simulink model "GRU_DataGen"  (R2024b)
settings: Solver=ode4  StartTime=0.0  StopTime=34  FixedStep=0.01  RelTol=1e-3
PreLoadFcn:
  | preloadfcn_v2
model workspace (MAT data in the model file):
  db_rt.A = [1 1 1 1 1 1 1 1 1 1 1 1 ... (55440 elements, 11x15x21x4x4)]
  db_rt.B = [0 0 0 0 0 0 0 0 -1.08359632143e-09 -1.08356536573e-09 -1.08354493529e-09 0 ... (27720 elements, 11x15x21x4x2)]
  db_rt.C = [1 1 1 1 1 1 1 1 1 1 1 1 ... (55440 elements, 11x15x21x4x4)]
  db_rt.D = [0 0 0 0 0 0 0 0 0 0 0 0 ... (27720 elements, 11x15x21x4x2)]
  db_rt.E = [3.5162966917e-06 3.51629595104e-06 2.9967648165e-06 2.99676418585e-06 2.9967635552e-06 2.99676229391e-06 2.99676040198e-06 2.99675567214e-06 4.11715267907e-06 4.11708414824e-06 4.11704028806e-06 3.00600683278e-06 ... (13860 elements, 11x15x21x4)]
  db_rt.grid.V = [0.02; 0.04; 0.06; 0.08; 0.1; 0.14; 0.2; 0.35; 0.6; 1; 1.2]
  db_rt.grid.W = [-1.2; -1.02857142857; -0.857142857143; -0.685714285714; -0.514285714286; -0.342857142857; -0.171428571429; 0; 0.171428571429; 0.342857142857; 0.514285714286; 0.685714285714; 0.857142857143; 1.02857142857; 1.2]
  db_rt.grid.T = [-0.174532925199; -0.157079632679; -0.13962634016; -0.12217304764; -0.10471975512; -0.0872664625997; -0.0698131700798; -0.0523598775598; -0.0349065850399; -0.0174532925199; 0; 0.0174532925199; 0.0349065850399; 0.0523598775598; 0.0698131700798; 0.0872664625997; 0.10471975512; 0.12217304764; 0.13962634016; 0.157079632679; 0.174532925199]
  db_rt.Ts = 0.01
  db_rt.nx = 4
  db_rt.nu = 2
  db_rt.ny = 4
  db_rt.nd = 1
  db_rt.Nv = 11
  db_rt.Nw = 15
  db_rt.Nt = 21
  env_paths.root = 'E:\Matlab\Simulink\S-Function_16'
  env_paths.data = 'E:\Matlab\Simulink\S-Function_16\data'
  env_paths.models = 'E:\Matlab\Simulink\S-Function_16\data\models'
  env_paths.paths = 'E:\Matlab\Simulink\S-Function_16\data\paths'
  env_paths.gru = 'E:\Matlab\Simulink\S-Function_16\data\gru'
  env_paths.results.root = 'E:\Matlab\Simulink\S-Function_16\results'
  env_paths.results.simulink = 'E:\Matlab\Simulink\S-Function_16\results\simulink'
  env_paths.results.closed_loop = 'E:\Matlab\Simulink\S-Function_16\results\closed_loop'
  env_paths.results.paths = 'E:\Matlab\Simulink\S-Function_16\results\paths'
  env_paths.results.gru_logs = 'E:\Matlab\Simulink\S-Function_16\results\gru\sim'
  ff_rt.m = 200
  ff_rt.g = 9.81
  ff_rt.c_r = 0.015
  ff_rt.rho = 1.225
  ff_rt.CdA = 0.5
  params.Ts = 0.01
  params.mass = 200
  params.L = 2
  params.W = 0.8
  params.h_cg = 0.5
  params.Lf = 1
  params.Lr = 1
  params.Iz = 16.67
  params.wheel_radius = 0.15
  params.wheel_mass = 1.2
  params.wheel_inertia = 0.0135
  params.motor_torque_constant = 1.21
  params.motor_inertia = 0.00177
  params.motor_current_limit = 9
  params.gear_ratio = 10
  params.gear_efficiency = 0.9
  params.current_limit = 9
  params.steering_time_constant = 0.08
  params.max_steering_angle = 1.57079632679
  params.max_steering_rate = 0.523598775598
  params.max_acceleration = 1
  params.rolling_resistance = 0.015
  params.friction_coefficient = 0.8
  params.air_density = 1.225
  params.drag_coefficient_area = 0.5
  params.gravity = 9.81
  params.front_cornering_stiffness = 300
  params.rear_cornering_stiffness = 300
  params.enable_noise = 0
  params.current_noise_std = 0.2
  params.wheel_speed_noise_std = 0.5
  params.disturbance_noise_std = 3
  params.random_seed = 42
  params.v_noise_std = 0.05
  params.psi_noise_std = 0.00872664625997
  params.omega_noise_std = 0.01
  params.min_angular_velocity_threshold = 0.001
  params.low_speed_threshold = 0.05
  params.use_smooth_saturation = 0
  params.smooth_gain = 30
  params.initial_x = 0
  params.initial_y = 0
  params.initial_heading = 0
  params.initial_velocity = 0
  params.initial_angular_velocity = 0
  params.initial_front_steering = 0
  params.initial_rear_steering = 0
  params.initial_sideslip = 0
  params.ai_backend = 'tcp_service'
  params.ai_model_type = 'mamba2'
  params.ai_model_path = ''
  params.ai_model_meta_path = ''
  params.ai_infer_interval = 5
  params.version = 'V4.1'
  params.creation_date = '2026-04-24 20:17:21'
  results_paths.root = 'E:\Matlab\Simulink\S-Function_16\results'
  results_paths.simulink = 'E:\Matlab\Simulink\S-Function_16\results\simulink'
  results_paths.closed_loop = 'E:\Matlab\Simulink\S-Function_16\results\closed_loop'
  results_paths.paths = 'E:\Matlab\Simulink\S-Function_16\results\paths'
  results_paths.gru_logs = 'E:\Matlab\Simulink\S-Function_16\results\gru\sim'
  v_ff_nom = 1
undefined symbols (not defined in the file): MPC_idx
libraries: mpclib x2
settings Model: Creator=15754  LastModifiedBy=15754

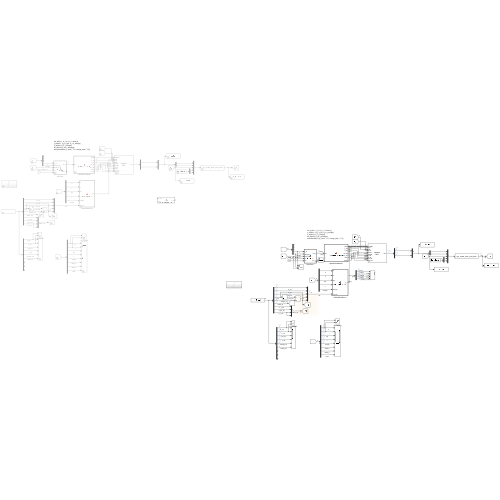
[thumbnail: Simulink's stored preview of the top-level diagram]
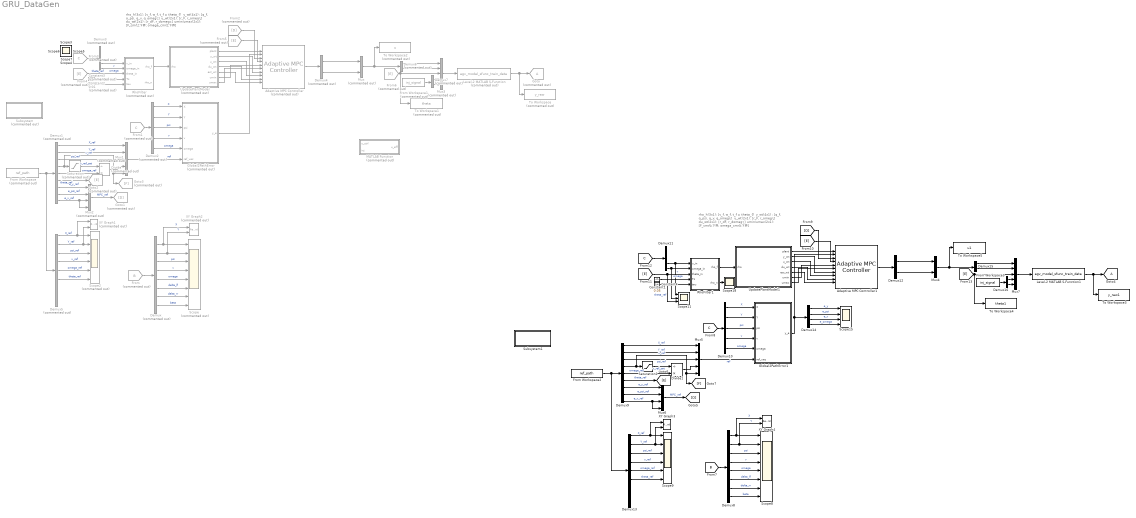
== system GRU_DataGen ==
  note: rho_h(3x1)：[v_f, w_f, t_f = theta_f]。
      | y_wt(4x1)：[q_f, q_psi, q_v, q_omega]。
      | u_wt(2x1): [r_F, r_omega]。
      | du_wt(2x1): [r_dF, r_domega]。
      | umin/umax(2x1): [F_cmd上下界; omega_cmd上下界]
  note: rho_h(3x1)：[v_f, w_f, t_f = theta_f]。
      | y_wt(4x1)：[q_f, q_psi, q_v, q_omega]。
      | u_wt(2x1): [r_F, r_omega]。
      | du_wt(2x1): [r_dF, r_domega]。
      | umin/umax(2x1): [F_cmd上下界; omega_cmd上下界]
  Adaptive MPC Controller : mpclib/Adaptive MPC Controller  Commented=on  SCDEnableBlockLinearizationSpecification=on  mpcobj=ctrl.mpcobj  enable_value=0  updateMPCinCallerWorkspace=on  md_inport=on  mv_inport=off  uref_inport=off  return_cost=off  return_mvseq=off  return_qpstatus=off  return_xseq=off  return_state=off  return_ovseq=off  state_inport=off  isltv_plant=off  umin_inport=on  umax_inport=on  ymin_inport=off  ymax_inport=off  cc_inport=off  ywt_inport=on  uwt_inport=on  duwt_inport=on  rhoeps_inport=on  pm_inport=off  MaximumP=10  HorizonChoice=FixedHorizon  BlockDataType=double  SampleTimeInherited=off  switch_inport=off
  Adaptive MPC Controller1 : mpclib/Adaptive MPC Controller  SCDEnableBlockLinearizationSpecification=on  mpcobj=ctrl.mpcobj  enable_value=0  updateMPCinCallerWorkspace=on  md_inport=on  mv_inport=off  uref_inport=off  return_cost=off  return_mvseq=off  return_qpstatus=off  return_xseq=off  return_state=off  return_ovseq=off  state_inport=off  isltv_plant=off  umin_inport=on  umax_inport=on  ymin_inport=off  ymax_inport=off  cc_inport=off  ywt_inport=on  uwt_inport=on  duwt_inport=on  rhoeps_inport=on  pm_inport=off  MaximumP=10  HorizonChoice=FixedHorizon  BlockDataType=double  SampleTimeInherited=off  switch_inport=off
  Constant1 : Constant  Value=0.05  SampleTime=params.Ts
  Constant2 : Constant  Commented=on  Value=0.01  SampleTime=params.Ts
  Constant3 : Constant  Commented=on  Value=0.4  SampleTime=params.Ts
  Constant4 : Constant  Value=0.4  SampleTime=params.Ts
  Demux : Demux  Commented=on  Outputs=8
  Demux1 : Demux  Commented=on  Outputs=9
  Demux10 : Demux  Outputs=5
  Demux11 : Demux  Outputs=5
  Demux12 : Demux  Outputs=2
  Demux13 : Demux  Outputs=9
  Demux14 : Demux
  Demux15 : Demux  Outputs=2
  Demux16 : Demux  Outputs=2
  Demux2 : Demux  Commented=on  Outputs=5
  Demux3 : Demux  Commented=on  Outputs=5
  Demux4 : Demux  Commented=on  Outputs=2
  Demux5 : Demux  Commented=on  Outputs=9
  Demux6 : Demux  Commented=on  Outputs=2
  Demux7 : Demux  Commented=on  Outputs=2
  Demux8 : Demux  Outputs=8
  Demux9 : Demux  Outputs=9
  Divide : Product  Commented=on  Inputs=/*
  Divide1 : Product  Inputs=/*
  From : From  Commented=on  GotoTag=B  TagVisibility=global
  From Workspace : FromWorkspace  Commented=on  VariableName=ref_path  SampleTime=params.Ts
  From Workspace1 : FromWorkspace  Commented=on  VariableName=inj_signal  SampleTime=params.Ts
  From Workspace2 : FromWorkspace  VariableName=ref_path  SampleTime=params.Ts
  From Workspace3 : FromWorkspace  VariableName=inj_signal  SampleTime=params.Ts
  From1 : From  Commented=on  GotoTag=C  TagVisibility=global
  From2 : From  Commented=on  GotoTag=D
  From3 : From  Commented=on  GotoTag=C  TagVisibility=global
  From4 : From  Commented=on  GotoTag=E
  From5 : From  Commented=on  GotoTag=E
  From6 : From  Commented=on  GotoTag=E
  Global2PathError : MATLAB Function  Commented=on  TreatAsAtomicUnit=on  SystemSampleTime=params.Ts
  Global2PathError1 : MATLAB Function  TreatAsAtomicUnit=on  SystemSampleTime=params.Ts
  Goto : Goto  Commented=on  TagVisibility=global
  Goto1 : Goto  Commented=on  GotoTag=D
  Goto2 : Goto  Commented=on  GotoTag=E
  Goto3 : Goto  Commented=on  GotoTag=F
  Goto4 : Goto  TagVisibility=global
  Level-2 MATLAB S-Function : M-S-Function  Commented=on  FunctionName=agv_model_sfunc_train_data  Parameters=parameters
  Level-2 MATLAB S-Function1 : M-S-Function  FunctionName=agv_model_sfunc_train_data  Parameters=parameters
  MATLAB Function : MATLAB Function  Commented=on  TreatAsAtomicUnit=on
  Mux : Mux  Commented=on  Inputs=2
  Mux1 : Mux  Commented=on  Inputs=5
  Mux2 : Mux  Commented=on
  Mux3 : Mux  Commented=on  Inputs=5
  Mux4 : Mux  Inputs=2
  Mux5 : Mux  Inputs=5
  Mux6 : Mux
  Mux7 : Mux  Inputs=5
  RhoFilter : MATLAB Function  Commented=on  TreatAsAtomicUnit=on
  RhoFilter1 : MATLAB Function  TreatAsAtomicUnit=on  SystemSampleTime=0.05
  Saturation : Saturate  Commented=on  UpperLimit=Inf  LowerLimit=1e-3
  Saturation1 : Saturate  UpperLimit=Inf  LowerLimit=1e-3
  Scope : Scope  Commented=on  NumInputPorts=8
  Scope11 : Scope  NumInputPorts=3
  Scope15 : Scope  NumInputPorts=4
  Scope{1,3..7,18} (7 alike) : Scope
  Scope2 : Scope  Commented=on  NumInputPorts=6
  Scope8 : Scope  NumInputPorts=8
  Scope9 : Scope  NumInputPorts=6
  Subsystem : Subsystem  Commented=on
  Subsystem1 : Subsystem
  To Workspace : ToWorkspace  Commented=on  VariableName=y_raw  SaveFormat=Structure With Time  SampleTime=params.Ts
  To Workspace1 : ToWorkspace  Commented=on  VariableName=theta  SaveFormat=Structure With Time  SampleTime=params.Ts
  To Workspace2 : ToWorkspace  Commented=on  VariableName=u  SaveFormat=Structure With Time  SampleTime=params.Ts
  To Workspace3 : ToWorkspace  VariableName=y_raw1  SaveFormat=Structure With Time  SampleTime=params.Ts
  To Workspace4 : ToWorkspace  VariableName=theta1  SaveFormat=Structure With Time  SampleTime=params.Ts
  To Workspace5 : ToWorkspace  VariableName=u1  SaveFormat=Structure With Time  SampleTime=params.Ts
  UpdatePlantModel : MATLAB Function  Commented=on  TreatAsAtomicUnit=on
  UpdatePlantModel1 : MATLAB Function  TreatAsAtomicUnit=on
  XY Graph1 : Record  Commented=on  FileSettingsInternal="{\"entries\":[{\"content\":{\"excelSettings\":{\"content\":{},\"type\":\"Streamout.ExcelSettings\"}},\"type\":\"Streamout.FileSettingStorage\",\"uuid\":\"\"}],\"packageUris\":[\"http:\\/\\/schema.mathworks.com\\/mf0\\/streamout_blocks\\/R2020a\"],\"version\":\"1.0\"}"  Layout=[1 1]  SignalsInternal="{\"entries\":[{\"content\":{\"signals\":[{\"content\":{\"blockPath\":[],\"dimensions\":[1],\"domain\":\"\",\"lineColor\":\"#edb120\",\"lineWidth\":2,\"port\":1,\"signalID\":1,\"signalName\":\"X_ref\"},\"type\":\"RecordBlkView.Signal\",\"uuid\":\"\"},{\"content\":{\"blockPath\":[],\"dimensions\":[1],\"domain\":\"\",\"lineColor\":\"#7e2f8e\",\"lineWidth\":2,\"port\":2,\"signalID\":2,\"signalName\":\"Y_ref\"},\"type\":\"RecordBlkView.Signal\",\"uuid\":\"\"}]},\"type\":\"RecordBlkView.InputSignals\",\"uuid\":\"\"}],\"packageUris\":[\"http:\\/\\/schema.mathworks.com\\/mf0\\/streamout_blocks\\/R2020a\"],\"version\":\"1.0\"}"  VisualizationBindings="{\"xyplotplugin\":{\"info\":[{\"series\":[],\"subplotID\":1}]}}"  CompatibilityTag=XY
  XY Graph2 : Record  Commented=on  FileSettingsInternal="{\"entries\":[{\"content\":{\"excelSettings\":{\"content\":{},\"type\":\"Streamout.ExcelSettings\"}},\"type\":\"Streamout.FileSettingStorage\",\"uuid\":\"\"}],\"packageUris\":[\"http:\\/\\/schema.mathworks.com\\/mf0\\/streamout_blocks\\/R2020a\"],\"version\":\"1.0\"}"  Layout=[1 1]  SignalsInternal="{\"entries\":[{\"content\":{\"signals\":[{\"content\":{\"blockPath\":[],\"dimensions\":[1],\"domain\":\"\",\"lineColor\":\"#b746ff\",\"lineWidth\":2,\"port\":1,\"signalID\":1,\"signalName\":\"X\"},\"type\":\"RecordBlkView.Signal\",\"uuid\":\"\"},{\"content\":{\"blockPath\":[],\"dimensions\":[1],\"domain\":\"\",\"lineColor\":\"#64d413\",\"lineWidth\":2,\"port\":2,\"signalID\":2,\"signalName\":\"Y\"},\"type\":\"RecordBlkView.Signal\",\"uuid\":\"\"}]},\"type\":\"RecordBlkView.InputSignals\",\"uuid\":\"\"}],\"packageUris\":[\"http:\\/\\/schema.mathworks.com\\/mf0\\/streamout_blocks\\/R2020a\"],\"version\":\"1.0\"}"  VisualizationBindings="{\"xyplotplugin\":{\"info\":[{\"series\":[],\"subplotID\":1}]}}"  CompatibilityTag=XY
  XY Graph3 : Record  FileSettingsInternal="{\"entries\":[{\"content\":{\"excelSettings\":{\"content\":{},\"type\":\"Streamout.ExcelSettings\"}},\"type\":\"Streamout.FileSettingStorage\",\"uuid\":\"\"}],\"packageUris\":[\"http:\\/\\/schema.mathworks.com\\/mf0\\/streamout_blocks\\/R2020a\"],\"version\":\"1.0\"}"  Layout=[1 1]  SignalsInternal="{\"entries\":[{\"content\":{\"signals\":[{\"content\":{\"blockPath\":[],\"dimensions\":[1],\"domain\":\"\",\"lineColor\":\"#a2142f\",\"plots\":[ 1 ],\"port\":1,\"sid\":[\"\"],\"signalID\":1,\"signalName\":\"X_ref\"},\"type\":\"RecordBlkView.Signal\",\"uuid\":\"\"},{\"content\":{\"blockPath\":[],\"dimensions\":[1],\"domain\":\"\",\"lineColor\":\"#139fff\",\"plots\":[ 1 ],\"port\":2,\"sid\":[\"\"],\"signalID\":2,\"signalName\":\"Y_ref\"},\"type\":\"RecordBlkView.Signal\",\"uuid\":\"\"}]},\"type\":\"RecordBlkView.InputSignals\",\"uuid\":\"\"}],\"packageUris\":[\"http:\\/\\/schema.mathworks.com\\/mf0\\/streamout_blocks\\/R2020a\"],\"version\":\"1.0\"}"  VisualizationBindings="{\"xyplotplugin\":{\"info\":[{\"series\":[{\"bindingParametersList\":[{\"parameter\":\"X-Axis\",\"signalID\":1,\"signalName\":\"X_ref\"},{\"parameter\":\"Y-Axis\",\"signalID\":2,\"signalName\":\"Y_ref\"}],\"seriesID\":0}],\"subplotID\":1}]}}"  CompatibilityTag=XY
  XY Graph4 : Record  FileSettingsInternal="{\"entries\":[{\"content\":{\"excelSettings\":{\"content\":{},\"type\":\"Streamout.ExcelSettings\"}},\"type\":\"Streamout.FileSettingStorage\",\"uuid\":\"\"}],\"packageUris\":[\"http:\\/\\/schema.mathworks.com\\/mf0\\/streamout_blocks\\/R2020a\"],\"version\":\"1.0\"}"  Layout=[1 1]  SignalsInternal="{\"entries\":[{\"content\":{\"signals\":[{\"content\":{\"blockPath\":[],\"dimensions\":[1],\"domain\":\"\",\"lineColor\":\"#a2142f\",\"plots\":[ 1 ],\"port\":1,\"sid\":[\"\"],\"signalID\":1,\"signalName\":\"X\"},\"type\":\"RecordBlkView.Signal\",\"uuid\":\"\"},{\"content\":{\"blockPath\":[],\"dimensions\":[1],\"domain\":\"\",\"lineColor\":\"#139fff\",\"plots\":[ 1 ],\"port\":2,\"sid\":[\"\"],\"signalID\":2,\"signalName\":\"Y\"},\"type\":\"RecordBlkView.Signal\",\"uuid\":\"\"}]},\"type\":\"RecordBlkView.InputSignals\",\"uuid\":\"\"}],\"packageUris\":[\"http:\\/\\/schema.mathworks.com\\/mf0\\/streamout_blocks\\/R2020a\"],\"version\":\"1.0\"}"  VisualizationBindings="{\"xyplotplugin\":{\"info\":[{\"series\":[{\"bindingParametersList\":[{\"parameter\":\"X-Axis\",\"signalID\":1,\"signalName\":\"X\"},{\"parameter\":\"Y-Axis\",\"signalID\":2,\"signalName\":\"Y\"}],\"seriesID\":0}],\"subplotID\":1}]}}"  CompatibilityTag=XY
  wires:
  Level-2 MATLAB S-Function/1 -> To Workspace/1, Goto/1
  From/1 -> Demux/1
  Demux/1 -> XY Graph2/1, Scope/1  "X"
  Demux/2 -> XY Graph2/2, Scope/2  "Y"
  Demux/3 -> Scope/3  "psi"
  Demux/4 -> Scope/4  "v"
  Demux/5 -> Scope/5  "omega"
  Demux/6 -> Scope/6  "delta_lf"
  Demux/7 -> Scope/7  "delta_rr"
  Demux/8 -> Scope/8  "beta"
  From Workspace/1 -> Demux5/1, Demux1/1
  Demux1/4 -> Goto3/1, Mux1/5, Saturation/1  "v_ref"
  Saturation/1 -> Divide/1  "v_ref_sat"
  Demux1/5 -> Divide/2  "omega_ref"
  Demux1/1 -> Mux1/1  "X_ref"
  Demux1/2 -> Mux1/2  "Y_ref"
  Demux1/3 -> Mux1/3  "psi_ref"
  Divide/1 -> Mux1/4
  Mux1/1 -> Global2PathError/6(ref_vec)  "ref"
  From1/1 -> Demux2/1
  Demux2/3 -> Global2PathError/3(psi)  "psi"
  Demux2/4 -> Global2PathError/4(v)  "v"
  Demux2/5 -> Global2PathError/5(omega)  "omega"
  Demux2/2 -> Global2PathError/2(Y)  "Y"
  Demux2/1 -> Global2PathError/1(X)  "X"
  Demux1/8 -> Mux2/2  "e_psi_ref"
  Demux1/7 -> Mux2/1  "e_y_ref"
  Demux1/9 -> Mux2/4, Mux2/3  "e_v_ref"
  Mux2/1 -> Goto1/1  "MPC_ref"
  From2/1 -> Adaptive MPC Controller/3
  From3/1 -> Demux3/1
  Demux3/4 -> RhoFilter/1(v_in)  "v"
  Demux3/5 -> RhoFilter/2(omega_in)  "omega"
  Demux1/6 -> Goto2/1  "theta_ref"
  From4/1 -> RhoFilter/3(theta_in)  "theta_ref"
  Constant2/1 -> RhoFilter/4(Ts)
  Constant3/1 -> RhoFilter/5(tau)
  UpdatePlantModel/1(plant) -> Adaptive MPC Controller/1
  From5/1 -> Adaptive MPC Controller/4
  RhoFilter/1(rho_f) -> UpdatePlantModel/1(rho)
  Demux5/1 -> XY Graph1/1, Scope2/1  "X_ref"
  Demux5/2 -> XY Graph1/2, Scope2/2  "Y_ref"
  Demux5/3 -> Scope2/3  "psi_ref"
  Demux5/4 -> Scope2/4  "v_ref"
  Demux5/5 -> Scope2/5  "omega_ref"
  Demux5/6 -> Scope2/6  "theta_ref"
  UpdatePlantModel/6(umin) -> Adaptive MPC Controller/5
  UpdatePlantModel/7(umax) -> Adaptive MPC Controller/6
  UpdatePlantModel/2(y_wt) -> Adaptive MPC Controller/7
  UpdatePlantModel/3(u_wt) -> Adaptive MPC Controller/8
  UpdatePlantModel/4(du_wt) -> Adaptive MPC Controller/9
  UpdatePlantModel/5(ecr_wt) -> Adaptive MPC Controller/10
  Global2PathError/1(y_e) -> Adaptive MPC Controller/2
  Adaptive MPC Controller/1 -> Demux4/1
  From6/1 -> Mux3/3, To Workspace1/1
  Demux4/2 -> Mux/2
  Mux/1 -> To Workspace2/1, Demux6/1
  Mux3/1 -> Level-2 MATLAB S-Function/1
  Demux6/1 -> Mux3/1
  Demux6/2 -> Mux3/2
  Demux7/1 -> Mux3/4
  Demux7/2 -> Mux3/5
  From Workspace1/1 -> Demux7/1
  Demux4/1 -> Mux/1
  Demux13/1 -> XY Graph3/1, Scope9/1  "X_ref"
  Demux8/8 -> Scope8/8  "beta"
  RhoFilter1/1(rho_f) -> UpdatePlantModel1/1(rho)
  Demux10/5 -> Global2PathError1/5(omega)  "omega"
  Demux13/6 -> Scope9/6  "theta_ref"
  Demux9/9 -> Mux6/4, Mux6/3  "e_v_ref"
  Demux11/5 -> Scope11/2, RhoFilter1/2(omega_in)  "omega"
  Demux8/3 -> Scope8/3  "psi"
  Global2PathError1/1(y_e) -> Adaptive MPC Controller1/2, Demux14/1
  UpdatePlantModel1/5(ecr_wt) -> Adaptive MPC Controller1/10
  Demux8/6 -> Scope8/6  "delta_lf"
  Demux13/3 -> Scope9/3  "psi_ref"
  Demux11/4 -> Scope11/1, RhoFilter1/1(v_in)  "v"
  Mux6/1 -> [D]  "MPC_ref"
  Demux14/3 -> Scope15/3  "e_v"
  UpdatePlantModel1/6(umin) -> Adaptive MPC Controller1/5
  UpdatePlantModel1/4(du_wt) -> Adaptive MPC Controller1/9
  Demux10/4 -> Global2PathError1/4(v)  "v"
  Demux9/6 -> [E]  "theta_ref"
  Mux5/1 -> Global2PathError1/6(ref_vec)  "ref"
  Demux8/5 -> Scope8/5  "omega"
  UpdatePlantModel1/7(umax) -> Adaptive MPC Controller1/6
  [E] -> Adaptive MPC Controller1/4
  Demux10/2 -> Global2PathError1/2(Y)  "Y"
  Demux14/2 -> Scope15/2  "e_psi"
  Demux8/7 -> Scope8/7  "delta_rr"
  Demux9/4 -> [F], Mux5/5, Saturation1/1  "v_ref"
  [D] -> Adaptive MPC Controller1/3
  Demux8/1 -> XY Graph4/1, Scope8/1  "X"
  Demux9/1 -> Mux5/1  "X_ref"
  Demux13/5 -> Scope9/5  "omega_ref"
  UpdatePlantModel1/1(plant) -> Adaptive MPC Controller1/1
  Demux10/3 -> Global2PathError1/3(psi)  "psi"
  Demux10/1 -> Global2PathError1/1(X)  "X"
  [E] -> Scope11/3, RhoFilter1/3(theta_in)  "theta_ref"
  Demux14/4 -> Scope15/4  "e_omega"
  RhoFilter1/2(rho_n) -> Scope18/1
  UpdatePlantModel1/2(y_wt) -> Adaptive MPC Controller1/7
  Demux9/5 -> Divide1/2  "omega_ref"
  Demux13/2 -> XY Graph3/2, Scope9/2  "Y_ref"
  Demux9/7 -> Mux6/1  "e_y_ref"
  Demux13/4 -> Scope9/4  "v_ref"
  Demux8/4 -> Scope8/4  "v"
  [C] -> Demux11/1
  Demux9/3 -> Mux5/3  "psi_ref"
  Constant4/1 -> RhoFilter1/5(tau)
  Demux8/2 -> XY Graph4/2, Scope8/2  "Y"
  Divide1/1 -> Mux5/4
  Saturation1/1 -> Divide1/1  "v_ref_sat"
  From Workspace2/1 -> Demux13/1, Demux9/1
  [B] -> Demux8/1
  Demux14/1 -> Scope15/1  "e_y"
  Demux9/8 -> Mux6/2  "e_psi_ref"
  UpdatePlantModel1/3(u_wt) -> Adaptive MPC Controller1/8
  [C] -> Demux10/1
  Constant1/1 -> RhoFilter1/4(Ts)
  Demux9/2 -> Mux5/2  "Y_ref"
  Demux12/1 -> Mux4/1
  From Workspace3/1 -> Demux16/1
  Demux16/2 -> Mux7/5
  Demux16/1 -> Mux7/4
  Demux15/2 -> Mux7/2
  Demux15/1 -> Mux7/1
  Mux7/1 -> Level-2 MATLAB S-Function1/1
  Mux4/1 -> Demux15/1, To Workspace5/1
  Demux12/2 -> Mux4/2
  [E] -> To Workspace4/1, Mux7/3
  Adaptive MPC Controller1/1 -> Demux12/1
  Level-2 MATLAB S-Function1/1 -> Goto4/1, To Workspace3/1

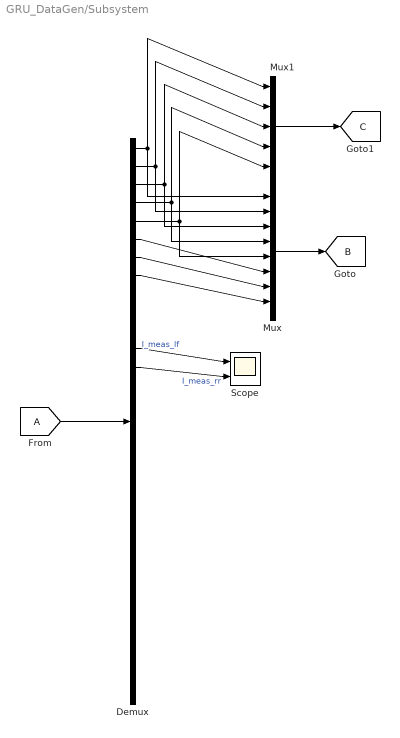
== system GRU_DataGen/Subsystem ==
  Demux : Demux  Outputs=31
  From : From  TagVisibility=global
  Mux : Mux  Inputs=8
  Mux1 : Mux  Inputs=5
  Scope : Scope  NumInputPorts=2
  tag scope: B=global, C=global
  wires:
  From/1 -> Demux/1
  Demux/1 -> Mux1/1, Mux/1
  Demux/2 -> Mux1/2, Mux/2
  Demux/3 -> Mux1/3, Mux/3
  Demux/4 -> Mux1/4, Mux/4
  Demux/5 -> Mux1/5, Mux/5
  Demux/6 -> Mux/6
  Demux/7 -> Mux/7
  Demux/8 -> Mux/8
  Mux/1 -> [B]
  Mux1/1 -> [C]
  Demux/12 -> Scope/1  "I_meas_lf"
  Demux/13 -> Scope/2  "I_meas_rr"

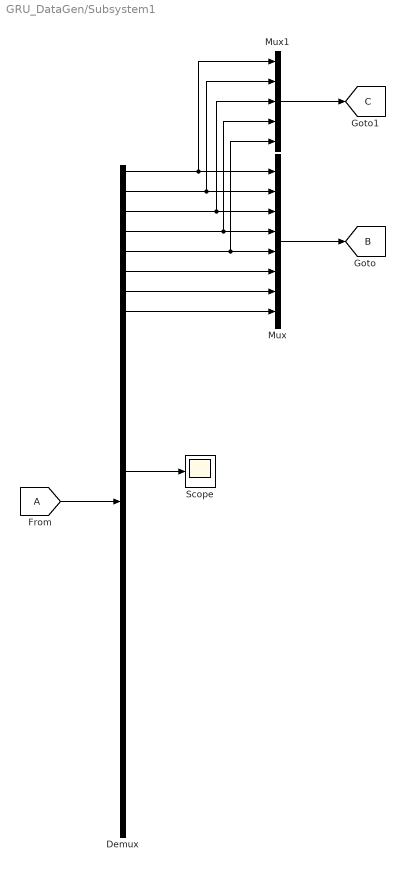
== system GRU_DataGen/Subsystem1 ==
  Demux : Demux  Outputs=34
  From : From  TagVisibility=global
  Mux : Mux  Inputs=8
  Mux1 : Mux  Inputs=5
  Scope : Scope
  tag scope: B=global, C=global
  wires:
  From/1 -> Demux/1
  Mux/1 -> [B]
  Mux1/1 -> [C]
  Demux/1 -> Mux/1, Mux1/1
  Demux/2 -> Mux1/2, Mux/2
  Demux/3 -> Mux1/3, Mux/3
  Demux/4 -> Mux1/4, Mux/4
  Demux/16 -> Scope/1
  Demux/5 -> Mux1/5, Mux/5
  Demux/6 -> Mux/6
  Demux/7 -> Mux/7
  Demux/8 -> Mux/8

== matlab function GRU_DataGen/UpdatePlantModel1 ==
  data: rho input; plant output Bus: MPCPlantBus; db_rt parameter; MPC_idx parameter double size=[1 4]; ff_rt parameter; v_ff_nom parameter; y_wt output; u_wt output; du_wt output; ecr_wt output; umin output; umax output
function [plant, y_wt, u_wt, du_wt, ecr_wt, umin, umax] = UpdatePlantModel(rho, db_rt, MPC_idx, ff_rt, v_ff_nom)
%#codegen
% =========================================================================
% UpdatePlantModel - 使用当前 phase1/phase2 最优参数 + Nominal 前馈
%
% 说明：
% 1) Q/R/dR 核心权重区间来自 phase1_best/phase2_best 的 best.ctrl_maps；
% 2) 场景自适应参数来自 phase2_best 的最新结果；
% 3) plant.U(1) 注入重力+滚阻前馈 F_eq，减小上坡“被惩罚”问题。
% =========================================================================

% 保留接口兼容
unused = MPC_idx; %#ok<NASGU>
unused = v_ff_nom; %#ok<NASGU>

%% ==================== 基于当前 BO 结果构建 maps_local ====================
% 当前读取来源：
% - Q/R/dR/rho范围/约束范围：phase2_best.mat -> best.ctrl_maps
% - 场景自适应参数：phase2_best.mat -> combined(best.ctrl_maps 同值)

Q_range_bo = [ ...
65.5231, 8.1684, 18.3989, 0.4160; ...
196.5693, 24.5051, 55.1966, 1.2481];

R_range_bo = [ ...
0.0015, 0.0058; ...
0.0046, 0.0173];

dR_range_bo = [ ...
0.0017, 0.1309; ...
0.0050, 0.3927];

maps_local = struct( ...
'enable_weight_interp', true, ...
'Q_range', Q_range_bo, ...
'R_range', R_range_bo, ...
'dR_range', dR_range_bo, ...
'alpha_Q', [0.5, 0.5, 0.5, 0.5], ...
'beta_Q', [0.5, 0.5, 0.5, 0.5], ...
'alpha_R', [0.5, 0.5], ...
'beta_R', [0.5, 0.5], ...
'alpha_dR', [0.5, 0.5], ...
'beta_dR', [0.5, 0.5], ...
'scale_umin_lo', [1, 1], ...
'scale_umin_hi', [1, 1], ...
'scale_umax_lo', [1, 1], ...
'scale_umax_hi', [1, 1], ...
'rho_min', [0.02; -1.2; -0.1745], ...
'rho_max', [1.2; 1.2; 0.1745], ...
'tau', 0.35, ...
'omega_threshold', 0.139817184968, ...
'q_y_gain_max', 5.54865433581, ...
'transition_width', 0.03, ...
'theta_threshold', 0.125151060428, ...
'q_v_gain_max', 3.46559044719, ...
'theta_transition_width', 0.02, ...
'R_F_gain_max_uphill', 1.00755999315, ...
'R_F_gain_max_downhill', 1.0, ...
'dR_F_gain_max_uphill', 1.0, ...
'dR_F_gain_max_downhill', 1.0, ...
'umin_range', [-720, -1.44; -600, -1.2], ...
'umax_range', [ 600, 1.2; 720, 1.44] ...
);

%% ==================== 在线插值：模型/权重/约束 ====================
upd = mpc_update_from_rho(rho, db_rt, maps_local);

%% ==================== 组装 plant（带 Nominal 前馈） ====================
nx = size(upd.A, 1);
ny = size(upd.C, 1);

plant.A = upd.A;

hasE = isfield(upd, 'E') && ~isempty(upd.E);
if hasE
E_col = upd.E;
else
E_col = zeros(nx, 1);
end

plant.B = [upd.B, E_col];
plant.C = upd.C;
plant.D = [upd.D, zeros(ny,1)];

% 重力 + 滚阻前馈
m_agv = ff_rt.m;
g_acc = ff_rt.g;
c_roll = ff_rt.c_r;
theta_meas = rho(3);

F_eq = m_agv * g_acc * (sin(theta_meas) + c_roll * cos(theta_meas));

% Nominal: [MV1; MV2; MD]
plant.U = [F_eq; 0; 0];
plant.X = zeros(nx,1);
plant.Y = zeros(ny,1);
plant.DX = zeros(nx,1);
plant.Ts = db_rt.Ts;

%% ==================== 输出给 MPC ====================
y_wt = upd.Q(:);
u_wt = upd.R(:);
du_wt = upd.dR(:);

ecr_wt = 1e4;
umin = upd.umin(:);
umax = upd.umax(:);

end

== matlab function GRU_DataGen/RhoFilter ==
  data: v_in input; rho_f output; omega_in input; theta_in input; Ts input; tau input; rho_n output
function [rho_f, rho_n] = RhoFilter(v_in, omega_in, theta_in, Ts, tau)
% 一阶离散滤波
persistent v_f_prev w_f_prev t_f_prev
if isempty(v_f_prev), v_f_prev = 0; end
if isempty(w_f_prev), w_f_prev = 0; end
if isempty(t_f_prev), t_f_prev = 0; end

a = Ts / max(tau + Ts, 1e-6);

v_f = (1 - a)*v_f_prev + a*max(v_in, 0);   % 速度不取负
w_f = (1 - a)*w_f_prev + a*omega_in;       % 保留符号
t_f = (1 - a)*t_f_prev + a*theta_in;       % 保留符号

v_f_prev = v_f; w_f_prev = w_f; t_f_prev = t_f;

rho_f = [v_f; w_f; t_f];

% 可选归一化（仅用于监控/调试，不参与UpdatePlantModel）
Vmax = 2.0; Wmax = 0.8; Tmax = deg2rad(10);
rho_n = [min(v_f/Vmax,1); min(abs(w_f)/Wmax,1); min(abs(t_f)/Tmax,1)];
end

== matlab function GRU_DataGen/Global2PathError ==
  data: X input; y_e output; Y input; psi input; v input; omega input; ref_vec input
% 误差计算模块
function y_e = Global2PathError(X, Y, psi, v, omega, ref_vec)
% ref_vec = [X_ref; Y_ref; psi_ref; kappa_ref; v_ref]
% 输出: y_e = [e_y; e_psi; e_v; e_omega; e_s]

%#codegen
% 1) 解包参考
Xr = ref_vec(1);
Yr = ref_vec(2);
psir = ref_vec(3);
kappa = ref_vec(4);
v_ref = ref_vec(5);

% 2) 横向误差：沿参考法向量投影（带符号）
ex = X - Xr; 
ey = Y - Yr;
e_y = -sin(psir)*ex + cos(psir)*ey;

% 3) 航向、速度、角速度误差
e_psi   = wrapToPi(psi - psir);
e_v     = v - v_ref;
omega_ff= v_ref * kappa;           % 曲率前馈
e_omega = omega - omega_ff;

% 4) 进度误差（可选，如未使用可置 0）
e_s = 0;

y_e = [e_y; e_psi; e_v; e_omega];
end

== matlab function GRU_DataGen/UpdatePlantModel ==
  data: rho input; plant output Bus: MPCPlantBus; db_rt parameter; MPC_idx parameter double size=[1 4]; ff_rt parameter; v_ff_nom parameter; y_wt output; u_wt output; du_wt output; ecr_wt output; umin output; umax output
function [plant, y_wt, u_wt, du_wt, ecr_wt, umin, umax] = UpdatePlantModel(rho, db_rt, MPC_idx, ff_rt, v_ff_nom)
%#codegen
% =========================================================================
% UpdatePlantModel - 使用当前 phase1/phase2 最优参数 + Nominal 前馈
%
% 说明：
% 1) Q/R/dR 核心权重区间来自 phase1_best/phase2_best 的 best.ctrl_maps；
% 2) 场景自适应参数来自 phase2_best 的最新结果；
% 3) plant.U(1) 注入重力+滚阻前馈 F_eq，减小上坡“被惩罚”问题。
% =========================================================================

% 保留接口兼容
unused = MPC_idx; %#ok<NASGU>
unused = v_ff_nom; %#ok<NASGU>

%% ==================== 基于当前 BO 结果构建 maps_local ====================
% 当前读取来源：
% - Q/R/dR/rho范围/约束范围：phase2_best.mat -> best.ctrl_maps
% - 场景自适应参数：phase2_best.mat -> combined(best.ctrl_maps 同值)

Q_range_bo = [ ...
65.5231, 8.1684, 18.3989, 0.4160; ...
196.5693, 24.5051, 55.1966, 1.2481];

R_range_bo = [ ...
0.0015, 0.0058; ...
0.0046, 0.0173];

dR_range_bo = [ ...
0.0017, 0.1309; ...
0.0050, 0.3927];

maps_local = struct( ...
'enable_weight_interp', true, ...
'Q_range', Q_range_bo, ...
'R_range', R_range_bo, ...
'dR_range', dR_range_bo, ...
'alpha_Q', [0.5, 0.5, 0.5, 0.5], ...
'beta_Q', [0.5, 0.5, 0.5, 0.5], ...
'alpha_R', [0.5, 0.5], ...
'beta_R', [0.5, 0.5], ...
'alpha_dR', [0.5, 0.5], ...
'beta_dR', [0.5, 0.5], ...
'scale_umin_lo', [1, 1], ...
'scale_umin_hi', [1, 1], ...
'scale_umax_lo', [1, 1], ...
'scale_umax_hi', [1, 1], ...
'rho_min', [0.02; -1.2; -0.1745], ...
'rho_max', [1.2; 1.2; 0.1745], ...
'tau', 0.35, ...
'omega_threshold', 0.139817184968, ...
'q_y_gain_max', 5.54865433581, ...
'transition_width', 0.03, ...
'theta_threshold', 0.125151060428, ...
'q_v_gain_max', 3.46559044719, ...
'theta_transition_width', 0.02, ...
'R_F_gain_max_uphill', 1.00755999315, ...
'R_F_gain_max_downhill', 1.0, ...
'dR_F_gain_max_uphill', 1.0, ...
'dR_F_gain_max_downhill', 1.0, ...
'umin_range', [-720, -1.44; -600, -1.2], ...
'umax_range', [ 600, 1.2; 720, 1.44] ...
);

%% ==================== 在线插值：模型/权重/约束 ====================
upd = mpc_update_from_rho(rho, db_rt, maps_local);

%% ==================== 组装 plant（带 Nominal 前馈） ====================
nx = size(upd.A, 1);
ny = size(upd.C, 1);

plant.A = upd.A;

hasE = isfield(upd, 'E') && ~isempty(upd.E);
if hasE
E_col = upd.E;
else
E_col = zeros(nx, 1);
end

plant.B = [upd.B, E_col];
plant.C = upd.C;
plant.D = [upd.D, zeros(ny,1)];

% 重力 + 滚阻前馈
m_agv = ff_rt.m;
g_acc = ff_rt.g;
c_roll = ff_rt.c_r;
theta_meas = rho(3);

F_eq = m_agv * g_acc * (sin(theta_meas) + c_roll * cos(theta_meas));

% Nominal: [MV1; MV2; MD]
plant.U = [F_eq; 0; 0];
plant.X = zeros(nx,1);
plant.Y = zeros(ny,1);
plant.DX = zeros(nx,1);
plant.Ts = db_rt.Ts;

%% ==================== 输出给 MPC ====================
y_wt = upd.Q(:);
u_wt = upd.R(:);
du_wt = upd.dR(:);

ecr_wt = 1e4;
umin = upd.umin(:);
umax = upd.umax(:);

end

== matlab function GRU_DataGen/Global2PathError1 ==
  data: X input; y_e output; Y input; psi input; v input; omega input; ref_vec input
% 误差计算模块
function y_e = Global2PathError(X, Y, psi, v, omega, ref_vec)
% ref_vec = [X_ref; Y_ref; psi_ref; kappa_ref; v_ref]
% 输出: y_e = [e_y; e_psi; e_v; e_omega; e_s]

%#codegen
% 1) 解包参考
Xr = ref_vec(1);
Yr = ref_vec(2);
psir = ref_vec(3);
kappa = ref_vec(4);
v_ref = ref_vec(5);

% 2) 横向误差：沿参考法向量投影（带符号）
ex = X - Xr; 
ey = Y - Yr;
e_y = -sin(psir)*ex + cos(psir)*ey;

% 3) 航向、速度、角速度误差
e_psi   = wrapToPi(psi - psir);
e_v     = v - v_ref;
omega_ff= v_ref * kappa;           % 曲率前馈
e_omega = omega - omega_ff;
% e_omega = omega_ff - omega;

% 4) 进度误差（可选，如未使用可置 0）
e_s = 0;

y_e = [e_y; e_psi; e_v; e_omega];
end

== matlab function GRU_DataGen/MATLAB Function ==
  data: u_ctrl input; u_eff output; inj input
function u_eff = InjectionWrapper(u_ctrl, inj)
% 打滑/堵转注入封装
% 输入:
%   u_ctrl: [2×1] = [F_cmd; omega_cmd]
%   inj   : [2×1] = [slip_gamma; stall_load]
%            slip_gamma = 1.0 正常，<1 打滑
%            stall_load = 0 正常，>0 堵转
% 输出:
%   u_eff : [2×1] = [F_eff; omega_eff]

F_cmd = u_ctrl(1);
omega_cmd = u_ctrl(2);

slip_gamma = inj(1);
stall_load = inj(2);

% 打滑：降低牵引效率
% 堵转：施加外部负载
F_eff = slip_gamma * F_cmd - stall_load;

% 角速度指令不修改（转弯侧滑无法通过简单方式模拟）
omega_eff = omega_cmd;

u_eff = [F_eff; omega_eff];
end

== matlab function GRU_DataGen/RhoFilter1 ==
  data: v_in input; rho_f output; omega_in input; theta_in input; Ts input; tau input; rho_n output
function [rho_f, rho_n] = RhoFilter(v_in, omega_in, theta_in, Ts, tau)
% 一阶离散滤波
persistent v_f_prev w_f_prev t_f_prev
if isempty(v_f_prev), v_f_prev = 0; end
if isempty(w_f_prev), w_f_prev = 0; end
if isempty(t_f_prev), t_f_prev = 0; end

a = Ts / max(tau + Ts, 1e-6);

v_f = (1 - a)*v_f_prev + a*max(v_in, 0);   % 速度不取负·
w_f = (1 - a)*w_f_prev + a*omega_in;       % 保留符号
t_f = (1 - a)*t_f_prev + a*theta_in;       % 保留符号

v_f_prev = v_f; w_f_prev = w_f; t_f_prev = t_f;

rho_f = [v_f; w_f; t_f];

% 可选归一化（仅用于监控/调试，不参与UpdatePlantModel）
Vmax = 2.0; Wmax = 0.8; Tmax = deg2rad(10);
rho_n = [min(v_f/Vmax,1); min(abs(w_f)/Wmax,1); min(abs(t_f)/Tmax,1)];
end
